simulink model "rpi_send_data"  (R2017a)
settings: Solver=VariableStepAuto  StartTime=0.0  StopTime=inf  RelTol=1e-3
libraries: raspberrypilib x1
settings Model: SimulationMode=external  Creator=WARA  LastModifiedBy=WARA

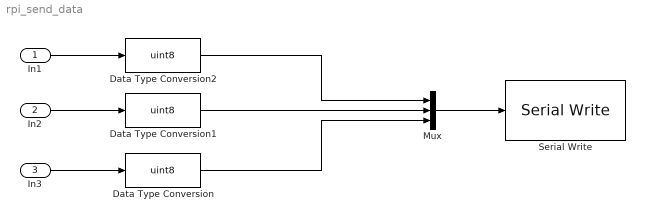
== system rpi_send_data ==
  In1 : Inport
  In2 : Inport  Port=2
  In3 : Inport  Port=3
  Data Type Conversion : DataTypeConversion  OutDataTypeStr=uint8
  Data Type Conversion1 : DataTypeConversion  OutDataTypeStr=uint8
  Data Type Conversion2 : DataTypeConversion  OutDataTypeStr=uint8
  Mux : Mux  Inputs=3
  Serial Write : raspberrypilib/Serial Write  board=Pi 3 Model B  SCIModule_=/dev/ttyS0  Baudrate_=9600  Parity=None  StopBits_=1  HardwareFlowControl=None  ByteOrder=LittleEndian  OutputStatus=off  blockPlatform=RaspberryPi
      settings: SourceProductName=Simulink Support Package for Raspberry Pi Hardware  SourceProductBaseCode=RASPPI
  wires:
  Data Type Conversion2/1 -> Mux/1
  Data Type Conversion/1 -> Mux/3
  Mux/1 -> Serial Write/1
  Data Type Conversion1/1 -> Mux/2
  In1/1 -> Data Type Conversion2/1
  In2/1 -> Data Type Conversion1/1
  In3/1 -> Data Type Conversion/1
